simulink model "Graficas_t1"  (R2024b)
settings: Solver=VariableStepAuto  StartTime=0.0  StopTime=10.0  RelTol=1e-3
settings Model: Creator=alexf  LastModifiedBy=alexf

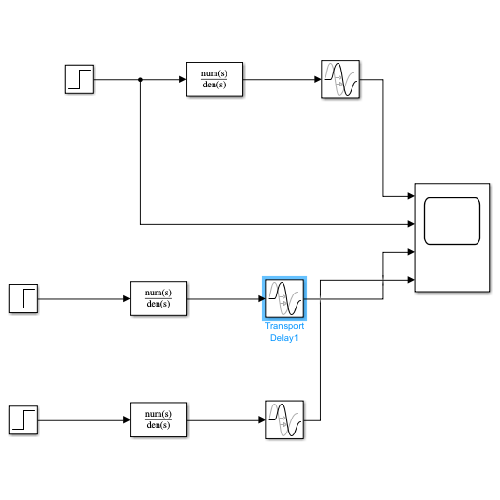
[thumbnail: Simulink's stored preview of the top-level diagram]
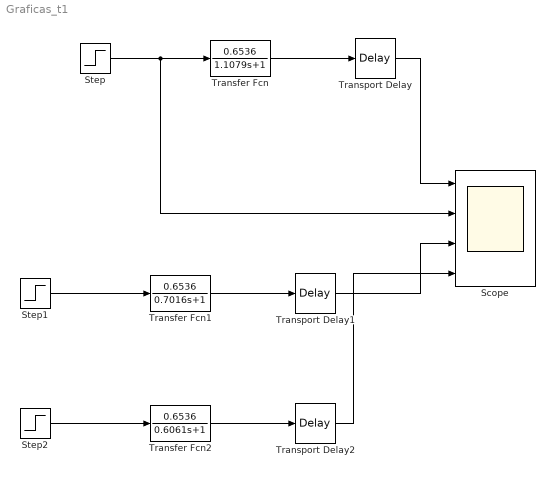
== system Graficas_t1 ==
  Scope : Scope  NumInputPorts=4
  Step : Step  Time=0.2020202  After=1.5  SampleTime=0
  Step1 : Step  Time=0.2020202  After=1.5  SampleTime=0
  Step2 : Step  Time=0.2020202  After=1.5  SampleTime=0
  Transfer Fcn : TransferFcn  Numerator=[0.6536]  Denominator=[1.1079 1]
  Transfer Fcn1 : TransferFcn  Numerator=[0.6536]  Denominator=[0.7016 1]
  Transfer Fcn2 : TransferFcn  Numerator=[0.6536]  Denominator=[0.6061 1]
  Transport Delay : TransportDelay  DelayTime=0.2784
  Transport Delay1 : TransportDelay  DelayTime=0.2784
  Transport Delay2 : TransportDelay  DelayTime=0.4040
  wires:
  Transport Delay/1 -> Scope/1
  Step/1 -> Transfer Fcn/1, Scope/2
  Transfer Fcn/1 -> Transport Delay/1
  Transfer Fcn1/1 -> Transport Delay1/1
  Step1/1 -> Transfer Fcn1/1
  Step2/1 -> Transfer Fcn2/1
  Transfer Fcn2/1 -> Transport Delay2/1
  Transport Delay1/1 -> Scope/3
  Transport Delay2/1 -> Scope/4
